simulink model "TestAttitudeControl"  (R2018b)
settings: Solver=VariableStepAuto  StartTime=0.0  StopTime=10  RelTol=1e-3
undefined symbols (not defined in the file): armed, ctrl_state, Initial, v_att_sp, v_control_mode
libraries: simulink_extras x2, simulink x1
(part 3 of 3)

== matlab function TestAttitudeControl/Euler Angles to Quaternion/MATLAB Function ==
  data: eulerAngles input; quat output
function quat   = EulerToQuaternion( eulerAngles )
%EULERTOQUATERNION Convert Euler angles to a quaternion
%   Based on PX4 Firmware code: https://github.com/PX4/Firmware
%   Written by: J.X.J. Bannwarth
%   Last modified: 29/08/2016

    roll  = eulerAngles(1);
    pitch = eulerAngles(2);
    yaw   = eulerAngles(3);

    cosPhi_2   = cos(roll / 2.0);
    sinPhi_2   = sin(roll / 2.0);
    cosTheta_2 = cos(pitch / 2.0);
    sinTheta_2 = sin(pitch / 2.0);
    cosPsi_2   = cos(yaw / 2.0);
    sinPsi_2   = sin(yaw / 2.0);

    quat = [ cosPhi_2 .* cosTheta_2 .* cosPsi_2 + sinPhi_2 .* sinTheta_2 .* sinPsi_2;
             sinPhi_2 .* cosTheta_2 .* cosPsi_2 - cosPhi_2 .* sinTheta_2 .* sinPsi_2;
             cosPhi_2 .* sinTheta_2 .* cosPsi_2 + sinPhi_2 .* cosTheta_2 .* sinPsi_2;
             cosPhi_2 .* cosTheta_2 .* sinPsi_2 - sinPhi_2 .* sinTheta_2 .* cosPsi_2 ];

end

== matlab function TestAttitudeControl/Quadrotor Quaternion Model/Quaternion to Rotation Matrix/MATLAB Function ==
  data: q input; R output
function R = QuatToRot( q )
%QUATTOROT Convert quaternion to rotation matrix
%   Written by:    J.X.J. Bannwarth, 2017/03/27
%   Last modified: J.X.J. Bannwarth, 2018/12/11
    W = q(1);
    X = q(2);
    Y = q(3);
    Z = q(4);
    
    xx = X * X;
    xy = X * Y;
    xz = X * Z;
    xw = X * W;

    yy = Y * Y;
    yz = Y * Z;
    yw = Y * W;
    
    zz = Z * Z;
    zw = Z * W;

    m00 = 1 - 2 * ( yy + zz );
    m01 =     2 * ( xy - zw );
    m02 =     2 * ( xz + yw );

    m10 =     2 * ( xy + zw );
    m11 = 1 - 2 * ( xx + zz );
    m12 =     2 * ( yz - xw );

    m20 =     2 * ( xz - yw );
    m21 =     2 * ( yz + xw );
    m22 = 1 - 2 * ( xx + yy );
    
    R = [m00 m01 m02;
         m10 m11 m12;
         m20 m21 m22];   
end

== matlab function TestAttitudeControl/Quadrotor Quaternion Model/Quaternion to Euler Angles/MATLAB Function ==
  data: quat input; eul output
function eul   = QuaternionToEuler( quat )
%QUATERNIONTOEULER Convert quaternion to euler angles
%   Based on PX4 Firmware code: https://github.com/PX4/Firmware
%   Written by:    J.X.J. Bannwarth, 2016/08/29
%   Last modified: J.X.J. Bannwarth, 2018/12/11

    eul = [ atan2(2.0 .* (quat(1) .* quat(2) + quat(3) .* quat(4)), ...
                1.0 - 2.0 .* (quat(2) .* quat(2) + quat(3) .* quat(3)));
	        asin(2.0 .* (quat(1) .* quat(3) - quat(4) .* quat(2)));
            atan2(2.0 .* (quat(1) .* quat(4) + quat(2) .* quat(3)), ...
                1.0 - 2.0 .* (quat(3) .* quat(3) + quat(4) .* quat(4))) ];
end
